simulink model "Mahalanobis"  (R2017a)
settings: Solver=VariableStepAuto  StartTime=0.0  StopTime=10.0  RelTol=1e-3
libraries: ad_blocks x10
settings Model: Creator=percro2  LastModifiedBy=percro2

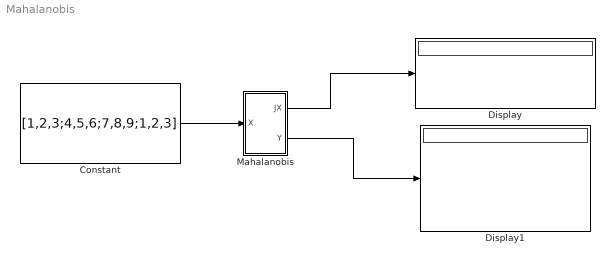
== system Mahalanobis ==
  Constant : Constant  Value=[1,2,3;4,5,6;7,8,9;1,2,3]  VectorParams1D=off
  Display : Display
  Display1 : Display
  Mahalanobis : Subsystem  mask{mu=[1,2,3;1,2,3;3,2,1;3,2,1], Sigma=[1,2,3,1;3,3,3,1;3,2,1,1;2,2,2,2]}
  wires:
  Constant/1 -> Mahalanobis/1(X)
  Mahalanobis/1(JX) -> Display/1
  Mahalanobis/2(Y) -> Display1/1

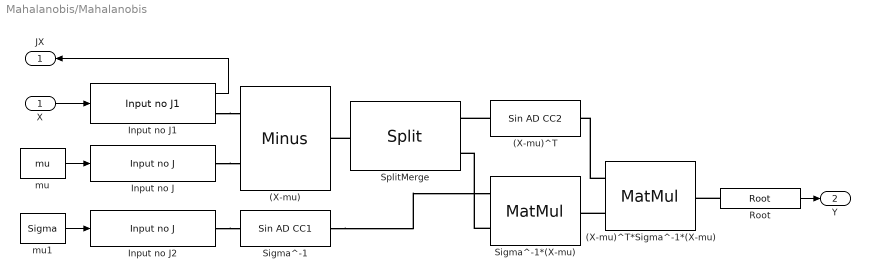
== system Mahalanobis/Mahalanobis ==
  X : Inport
  "(X-mu) " : ad_blocks/Minus   SystemSampleTime=-1
  (X-mu)^T : ad_blocks/Sin AD CC2  SystemSampleTime=-1
  (X-mu)^T*Sigma^-1*(X-mu) : ad_blocks/MatMul  SystemSampleTime=-1
  Input no J : ad_blocks/Input no J  SystemSampleTime=-1
  Input no J1 : ad_blocks/Input no J1  SystemSampleTime=-1
  Input no J2 : ad_blocks/Input no J  SystemSampleTime=-1
  Root : ad_blocks/Root  SystemSampleTime=-1
  Sigma^-1 : ad_blocks/Sin AD CC1  SystemSampleTime=-1
  Sigma^-1*(X-mu) : ad_blocks/MatMul  SystemSampleTime=-1
  SplitMerge : ad_blocks/Split  SystemSampleTime=-1
  mu : Constant  Value=mu  VectorParams1D=off
  mu1 : Constant  Value=Sigma  VectorParams1D=off
  JX : Outport
  Y : Outport  Port=2
  wires:
  X/1 -> Input no J1/1
  Root/1 -> Y/1
  Input no J1/1 -> JX/1
  mu/1 -> Input no J/1
  mu1/1 -> Input no J2/1
  connections:
  (X-mu)^T*Sigma^-1*(X-mu)/LConn2 -- Sigma^-1*(X-mu)/RConn1
  Input no J/RConn1 -- "(X-mu) "/LConn2
  Input no J1/RConn1 -- "(X-mu) "/LConn1
  SplitMerge/LConn1 -- "(X-mu) "/RConn1
  Sigma^-1*(X-mu)/LConn2 -- SplitMerge/RConn2
  Sigma^-1/RConn1 -- Sigma^-1*(X-mu)/LConn1
  Root/LConn1 -- (X-mu)^T*Sigma^-1*(X-mu)/RConn1
  (X-mu)^T*Sigma^-1*(X-mu)/LConn1 -- (X-mu)^T/RConn1
  Input no J2/RConn1 -- Sigma^-1/LConn1
  (X-mu)^T/LConn1 -- SplitMerge/RConn1
